simulink model "BicycleModel_MPC"  (R2022b)
settings: Solver=VariableStepAuto  StartTime=0.0  StopTime=19.3  RelTol=1e-3
model workspace: external: MATLAB File C:\Users\npn01\OneDrive - Mälardalens högskola\Desktop\Research\BPP\BicycleModelFillet\BicycleModelFillet_DataFile.m (data not in the file)
values from neighbouring files (symbols this model uses):
  bikepath = [refSpline(:,1), -refSpline(:,2) , refTheta]    [getRefPos.m]
undefined symbols (not defined in the file or in its folder): pidParam, Rd, simParams, smiData, trajSol, Ts, TsInner, X, Y, yOff, Z
libraries: sm_lib x201, nesl_utility x11, simulink x3, simulink_extras x3, slpidlib x1, fl_lib x1, mpclib x1
(part 5 of 5)

== system BicycleModel_MPC/Bicycle/Main frame/Frame_1_RIGID/Holder2_1_RIGID/U_Bolt_5_RIGID ==
  ReferenceFrame : sm_lib/Frames and Transforms/Reference Frame
  Solid : sm_lib/Body Elements/File Solid  ExtGeomFileName=U-Bolt_Motor_sldprt.STEP  UnitType=FromFile  ExtGeomFileUnits=m  StepReaderType=HEX  ExportConvexHullGeometry=off  InertiaType=Custom  Mass=smiData.Solid(11).mass  MassUnits=kg  CenterOfMass=smiData.Solid(11).CoM  CenterOfMassUnits=mm  MomentsOfInertia=smiData.Solid(11).MoI  MomentsOfInertiaUnits=kg*mm^2  ProductsOfInertia=smiData.Solid(11).PoI  ProductsOfInertiaUnits=kg*mm^2  BasedOnType=DensityFromFile  Density=1000  DensityUnits=kg/m^3  DoExposeReferenceFrame=on  SerializedFrames=<Frames/>  GraphicType=FromGeometry  MarkerShape=Sphere  MarkerSize=10  GraphicVisPropType=SimpleVisualProperties  GraphicDiffuseColor=smiData.Solid(11).color  GraphicSpecularColor=[0.5 0.5 0.5 1.0]  GraphicAmbientColor=[0.15 0.15 0.15 1.0]  GraphicEmissiveColor=[0.0 0.0 0.0 1.0]  GraphicShininess=75  GraphicOpacity=smiData.Solid(11).opacity
  F : PMIOPort  Side=Left
  connections:
  Solid/RConn1 -- ReferenceFrame/RConn1 -- F/RConn1

== matlab function BicycleModel_MPC/Subsystem/MATLAB Function ==
  data: simTime input; v output size=1; mpcV input
function v = fcn(simTime, mpcV)

if simTime > 0.5
    v = mpcV;
else
    if mpcV > 10
        v = 1.5 + 2 * simTime;
    else
        v = mpcV;
    end
end

== matlab function BicycleModel_MPC/Bicycle/Sense/quaternion to euler ==
  data: q input; roll output; yaw output
function [roll,yaw] = fcn(q)

siny_cosp = 2*(q(1)*q(4) + q(2)*q(3));
cosy_cosp = 1 - 2*(q(3)*q(3) + q(4)*q(4));
yaw = atan2(siny_cosp,cosy_cosp) ;
%yaw = atan2(sin(yaw), cos(yaw));

sinr_cosp = 2 * (q(1) * q(2) + q(3) * q(4));
cosr_cosp = 1 - 2 * (q(2) * q(2) + q(3) * q(3));
roll=atan2(sinr_cosp, cosr_cosp);

%roll=roll+pi;
roll=atan2(sin(roll),cos(roll));

== matlab function BicycleModel_MPC/Subsystem/Error reference/Time varying reference/Compute Ref ==
  data: currentPos input; ref output size=[20,20]; bikepath input; ref input; error output; PredictionHorizon input; refindex input
function [ref,error]   = ComputeRef(currentPos, bikepath, ref,PredictionHorizon, refindex)



PredictionHorizon = uint32(PredictionHorizon-1);
refindex =  uint32(refindex);
%Current position
currentPos = currentPos';

currentPos(1) = currentPos(1);
currentPos(3) = currentPos(3);


theta = currentPos(1);
xp = currentPos(2);
yp = currentPos(3);




%Extract the reference path, the length of the reference path will be equal
%to the prediction horizon

PathSegment=bikepath(refindex:refindex+PredictionHorizon, uint8([1 2 3 4 5]));

dx = 0;
dy = 0;
ephi   = 0;
edelta = 0;


for i = 1:PredictionHorizon+1
    %compute error
    error = PathSegment(i,:)-currentPos; %[theta, x, y, roll angle(phi)]
    etheta =  atan2(sin(error(1)),cos(error(1)));
    
    ex     = error(2);
    ey     = -error(3);
    % Compute variation in the bicycle frame
%         dx=cos(theta)*PathSegment(i,2) + sin(theta)*PathSegment(i,3);
%     dy=-sin(theta)*PathSegment(i,2) + cos(theta)*PathSegment(i,3);

%     dx=cos(theta-etheta)*ex + sin(theta-etheta)*ey;
% %     dy=-sin(theta-etheta)*ex + cos(theta-etheta)*ey;
%     testtheta = atan2( sin(theta - etheta), cos(theta-etheta));
%     
%     dx = cos( testtheta)*ex + sin( testtheta)*ey;
%     dy = -sin( testtheta)*ex + cos( testtheta)*ey;
%     dx = cos(theta-etheta)*ex + sin(theta-etheta)*ey;
%     dy = -sin(theta-etheta)*ex + cos(theta-etheta)*ey;
    dx = cos(theta)*ex + sin(theta)*ey;
    dy = -sin(theta)*ex + cos(theta)*ey;

    dtheta = etheta;
   % ref(i,:)= PathSegment(i,:)+[dtheta, dx, dy, 0, 0];
    ref(i,:) = [dtheta,dx,dy,ephi,edelta];
end 


%This outputs are just for debugging purpose
CurrentRef=bikepath(refindex,uint8([1 2 3 5])); %extract the current path (for plotting after simulation is done)
xy=[theta,xp,yp, CurrentRef(1:3)]; %<- this is plotted during the simulation


%For logging/debugging/plotting purpose
error=PathSegment(1,:)-currentPos; %[theta, x, y, roll angle(phi)]
etheta = atan2(sin(error(1)),cos(error(1)));
error=ref(1,:);



end

== matlab function BicycleModel_MPC/Bicycle/World/check ref ==
  data: xref output; bikepath input; yref output; refindex input; thetaref output
function [xref, yref, thetaref]   = GetCurrentRef(bikepath,refindex)


PathSegment = bikepath(refindex, uint8([1 2 3 4 5]));
xref = PathSegment(1,2);
yref = PathSegment(1,3);
thetaref = PathSegment(1,1);

end
